simulink model "asservrml"  (R2023a)
settings: Solver=VariableStepAuto  StartTime=0.0  StopTime=100  RelTol=1e-3
libraries: vrlib x5
settings Model: Creator=ayoub  LastModifiedBy=AI-MHT
settings SolverCC: AlgebraicLoopSolver=TrustRegion
settings DataIOCC: ReturnWorkspaceOutputs=off
settings DebuggingCC: UnconnectedInputMsg=warning  UnconnectedOutputMsg=warning  UnconnectedLineMsg=warning  ArithmeticOperatorsInVariantConditions=warning
settings ModelReferenceCC: EnableRefExpFcnMdlSchedulingChecks=on
settings SFSimCC: SimUseLocalCustomCode=off  CustomCodeUndefinedFunction=UseInterfaceOnly
settings RTWCC: RTWUseLocalCustomCode=off
settings CodeAppCC: StateflowObjectComments=on

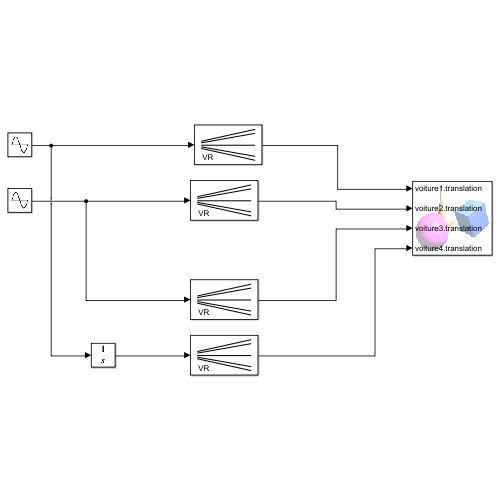
[thumbnail: Simulink's stored preview of the top-level diagram]
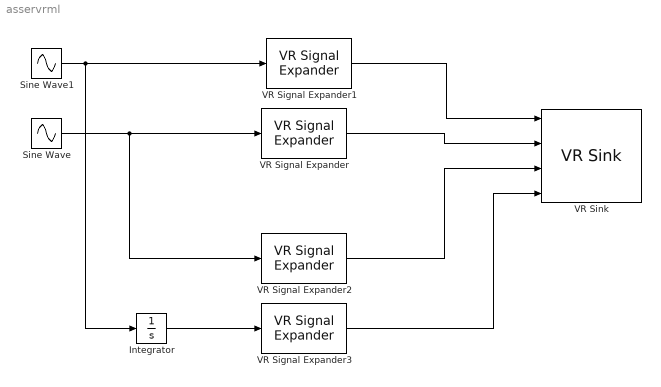
== system asservrml ==
  Integrator : Integrator
  Sine Wave : Sin  Amplitude=100  SampleTime=0
  Sine Wave1 : Sin  Amplitude=60  Frequency=0.8  Phase=30  SampleTime=0
  VR Signal Expander : vrlib/VR Signal Expander  outwidth=3  outidx=[1]
  VR Signal Expander1 : vrlib/VR Signal Expander  outwidth=3  outidx=[3]
  VR Signal Expander2 : vrlib/VR Signal Expander  outwidth=3  outidx=[3]
  VR Signal Expander3 : vrlib/VR Signal Expander  outwidth=3  outidx=[1]
  VR Sink : vrlib/VR Sink  InstantiateOnLoad=on  SampleTime=0.001  ViewEnable=on  RemoteChange=off  RemoteView=off  FieldsWritten=voiture1.translation.3.1.1.double#voiture2.translation.3.1.1.double#voiture3.translation.3.1.1.double#voiture4.translation.3.1.1.double  WorldFileName=carrefour3d.wrl  AutoView=off  VideoDimensions=[]  AllowVariableSize=off
  wires:
  Sine Wave/1 -> VR Signal Expander2/1, VR Signal Expander/1
  Sine Wave1/1 -> Integrator/1, VR Signal Expander1/1
  Integrator/1 -> VR Signal Expander3/1
  VR Signal Expander1/1 -> VR Sink/1
  VR Signal Expander/1 -> VR Sink/2
  VR Signal Expander2/1 -> VR Sink/3
  VR Signal Expander3/1 -> VR Sink/4
